simulink library "csc_tdl_thruster_dynamics_collection_lib"  (R2014b)
settings: Solver=ode45  StartTime=0.0  StopTime=10.0  RelTol=1e-3
libraries: csu_tdl_thruster_dynamics_lander_lib x26
settings Model: Creator=escrane  LastModifiedBy=mstewart

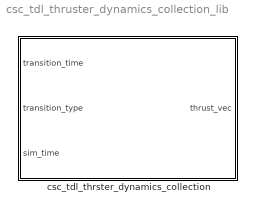
== system csc_tdl_thruster_dynamics_collection_lib ==
  csc_tdl_thrster_dynamics_collection : Subsystem
      mask Display: color('blue');text(0.05, 0.02, 'MoonEx', 'HorizontalAlignment', 'Left', 'VerticalAlignment', 'Bottom');color('red');text(0.95, 0.02, 'Autogenerated', 'HorizontalAlignment', 'Right', 'VerticalAlignment', 'Bottom');

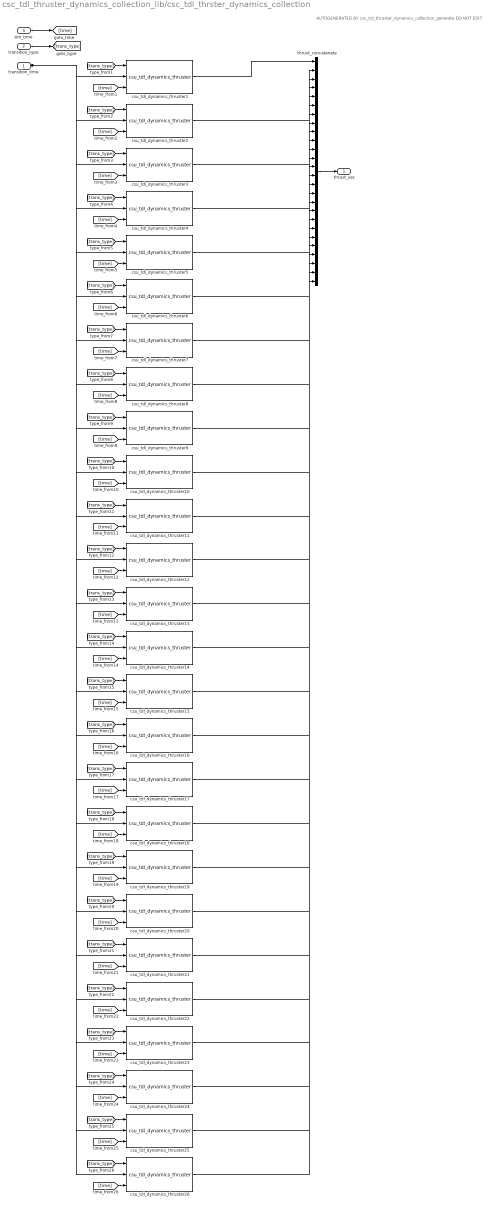
== system csc_tdl_thruster_dynamics_collection_lib/csc_tdl_thrster_dynamics_collection ==
  note: AUTOGENERATED BY csc_tdl_thruster_dynamics_collection_generate
      | DO NOT EDIT
  transition_time : Inport
  transition_type : Inport  Port=2
  sim_time : Inport  Port=3
  csu_tdl_dynamics_thruster1 : csu_tdl_thruster_dynamics_lander_lib/csu_tdl_dynamics_thruster  thruster_idx=1  num_thrusters=26  time_since_rise_lookup=tdl_thruster1_rising_lookup_time  thrust_rising_output_lookup=tdl_thruster1_rising_lookup_thrust  time_since_fall_lookup=tdl_thruster1_falling_lookup_time  thrust_falling_output_lookup=tdl_thruster1_falling_lookup_thrust  thrust_noise_mean=tdl_thruster1_thrust_noise_mean  thrust_noise_std=tdl_thruster1_thrust_noise_std  thrust_noise_seed=tdl_thruster1_thrust_noise_seed  thrust_noise_on=tdl_thruster1_thrust_noise_enable
  csu_tdl_dynamics_thruster10 : csu_tdl_thruster_dynamics_lander_lib/csu_tdl_dynamics_thruster  thruster_idx=10  num_thrusters=26  time_since_rise_lookup=tdl_thruster10_rising_lookup_time  thrust_rising_output_lookup=tdl_thruster10_rising_lookup_thrust  time_since_fall_lookup=tdl_thruster10_falling_lookup_time  thrust_falling_output_lookup=tdl_thruster10_falling_lookup_thrust  thrust_noise_mean=tdl_thruster10_thrust_noise_mean  thrust_noise_std=tdl_thruster10_thrust_noise_std  thrust_noise_seed=tdl_thruster10_thrust_noise_seed  thrust_noise_on=tdl_thruster10_thrust_noise_enable
  csu_tdl_dynamics_thruster11 : csu_tdl_thruster_dynamics_lander_lib/csu_tdl_dynamics_thruster  thruster_idx=11  num_thrusters=26  time_since_rise_lookup=tdl_thruster11_rising_lookup_time  thrust_rising_output_lookup=tdl_thruster11_rising_lookup_thrust  time_since_fall_lookup=tdl_thruster11_falling_lookup_time  thrust_falling_output_lookup=tdl_thruster11_falling_lookup_thrust  thrust_noise_mean=tdl_thruster11_thrust_noise_mean  thrust_noise_std=tdl_thruster11_thrust_noise_std  thrust_noise_seed=tdl_thruster11_thrust_noise_seed  thrust_noise_on=tdl_thruster11_thrust_noise_enable
  csu_tdl_dynamics_thruster12 : csu_tdl_thruster_dynamics_lander_lib/csu_tdl_dynamics_thruster  thruster_idx=12  num_thrusters=26  time_since_rise_lookup=tdl_thruster12_rising_lookup_time  thrust_rising_output_lookup=tdl_thruster12_rising_lookup_thrust  time_since_fall_lookup=tdl_thruster12_falling_lookup_time  thrust_falling_output_lookup=tdl_thruster12_falling_lookup_thrust  thrust_noise_mean=tdl_thruster12_thrust_noise_mean  thrust_noise_std=tdl_thruster12_thrust_noise_std  thrust_noise_seed=tdl_thruster12_thrust_noise_seed  thrust_noise_on=tdl_thruster12_thrust_noise_enable
  csu_tdl_dynamics_thruster13 : csu_tdl_thruster_dynamics_lander_lib/csu_tdl_dynamics_thruster  thruster_idx=13  num_thrusters=26  time_since_rise_lookup=tdl_thruster13_rising_lookup_time  thrust_rising_output_lookup=tdl_thruster13_rising_lookup_thrust  time_since_fall_lookup=tdl_thruster13_falling_lookup_time  thrust_falling_output_lookup=tdl_thruster13_falling_lookup_thrust  thrust_noise_mean=tdl_thruster13_thrust_noise_mean  thrust_noise_std=tdl_thruster13_thrust_noise_std  thrust_noise_seed=tdl_thruster13_thrust_noise_seed  thrust_noise_on=tdl_thruster13_thrust_noise_enable
  csu_tdl_dynamics_thruster14 : csu_tdl_thruster_dynamics_lander_lib/csu_tdl_dynamics_thruster  thruster_idx=14  num_thrusters=26  time_since_rise_lookup=tdl_thruster14_rising_lookup_time  thrust_rising_output_lookup=tdl_thruster14_rising_lookup_thrust  time_since_fall_lookup=tdl_thruster14_falling_lookup_time  thrust_falling_output_lookup=tdl_thruster14_falling_lookup_thrust  thrust_noise_mean=tdl_thruster14_thrust_noise_mean  thrust_noise_std=tdl_thruster14_thrust_noise_std  thrust_noise_seed=tdl_thruster14_thrust_noise_seed  thrust_noise_on=tdl_thruster14_thrust_noise_enable
  csu_tdl_dynamics_thruster15 : csu_tdl_thruster_dynamics_lander_lib/csu_tdl_dynamics_thruster  thruster_idx=15  num_thrusters=26  time_since_rise_lookup=tdl_thruster15_rising_lookup_time  thrust_rising_output_lookup=tdl_thruster15_rising_lookup_thrust  time_since_fall_lookup=tdl_thruster15_falling_lookup_time  thrust_falling_output_lookup=tdl_thruster15_falling_lookup_thrust  thrust_noise_mean=tdl_thruster15_thrust_noise_mean  thrust_noise_std=tdl_thruster15_thrust_noise_std  thrust_noise_seed=tdl_thruster15_thrust_noise_seed  thrust_noise_on=tdl_thruster15_thrust_noise_enable
  csu_tdl_dynamics_thruster16 : csu_tdl_thruster_dynamics_lander_lib/csu_tdl_dynamics_thruster  thruster_idx=16  num_thrusters=26  time_since_rise_lookup=tdl_thruster16_rising_lookup_time  thrust_rising_output_lookup=tdl_thruster16_rising_lookup_thrust  time_since_fall_lookup=tdl_thruster16_falling_lookup_time  thrust_falling_output_lookup=tdl_thruster16_falling_lookup_thrust  thrust_noise_mean=tdl_thruster16_thrust_noise_mean  thrust_noise_std=tdl_thruster16_thrust_noise_std  thrust_noise_seed=tdl_thruster16_thrust_noise_seed  thrust_noise_on=tdl_thruster16_thrust_noise_enable
  csu_tdl_dynamics_thruster17 : csu_tdl_thruster_dynamics_lander_lib/csu_tdl_dynamics_thruster  thruster_idx=17  num_thrusters=26  time_since_rise_lookup=tdl_thruster17_rising_lookup_time  thrust_rising_output_lookup=tdl_thruster17_rising_lookup_thrust  time_since_fall_lookup=tdl_thruster17_falling_lookup_time  thrust_falling_output_lookup=tdl_thruster17_falling_lookup_thrust  thrust_noise_mean=tdl_thruster17_thrust_noise_mean  thrust_noise_std=tdl_thruster17_thrust_noise_std  thrust_noise_seed=tdl_thruster17_thrust_noise_seed  thrust_noise_on=tdl_thruster17_thrust_noise_enable
  csu_tdl_dynamics_thruster18 : csu_tdl_thruster_dynamics_lander_lib/csu_tdl_dynamics_thruster  thruster_idx=18  num_thrusters=26  time_since_rise_lookup=tdl_thruster18_rising_lookup_time  thrust_rising_output_lookup=tdl_thruster18_rising_lookup_thrust  time_since_fall_lookup=tdl_thruster18_falling_lookup_time  thrust_falling_output_lookup=tdl_thruster18_falling_lookup_thrust  thrust_noise_mean=tdl_thruster18_thrust_noise_mean  thrust_noise_std=tdl_thruster18_thrust_noise_std  thrust_noise_seed=tdl_thruster18_thrust_noise_seed  thrust_noise_on=tdl_thruster18_thrust_noise_enable
  csu_tdl_dynamics_thruster19 : csu_tdl_thruster_dynamics_lander_lib/csu_tdl_dynamics_thruster  thruster_idx=19  num_thrusters=26  time_since_rise_lookup=tdl_thruster19_rising_lookup_time  thrust_rising_output_lookup=tdl_thruster19_rising_lookup_thrust  time_since_fall_lookup=tdl_thruster19_falling_lookup_time  thrust_falling_output_lookup=tdl_thruster19_falling_lookup_thrust  thrust_noise_mean=tdl_thruster19_thrust_noise_mean  thrust_noise_std=tdl_thruster19_thrust_noise_std  thrust_noise_seed=tdl_thruster19_thrust_noise_seed  thrust_noise_on=tdl_thruster19_thrust_noise_enable
  csu_tdl_dynamics_thruster2 : csu_tdl_thruster_dynamics_lander_lib/csu_tdl_dynamics_thruster  thruster_idx=2  num_thrusters=26  time_since_rise_lookup=tdl_thruster2_rising_lookup_time  thrust_rising_output_lookup=tdl_thruster2_rising_lookup_thrust  time_since_fall_lookup=tdl_thruster2_falling_lookup_time  thrust_falling_output_lookup=tdl_thruster2_falling_lookup_thrust  thrust_noise_mean=tdl_thruster2_thrust_noise_mean  thrust_noise_std=tdl_thruster2_thrust_noise_std  thrust_noise_seed=tdl_thruster2_thrust_noise_seed  thrust_noise_on=tdl_thruster2_thrust_noise_enable
  csu_tdl_dynamics_thruster20 : csu_tdl_thruster_dynamics_lander_lib/csu_tdl_dynamics_thruster  thruster_idx=20  num_thrusters=26  time_since_rise_lookup=tdl_thruster20_rising_lookup_time  thrust_rising_output_lookup=tdl_thruster20_rising_lookup_thrust  time_since_fall_lookup=tdl_thruster20_falling_lookup_time  thrust_falling_output_lookup=tdl_thruster20_falling_lookup_thrust  thrust_noise_mean=tdl_thruster20_thrust_noise_mean  thrust_noise_std=tdl_thruster20_thrust_noise_std  thrust_noise_seed=tdl_thruster20_thrust_noise_seed  thrust_noise_on=tdl_thruster20_thrust_noise_enable
  csu_tdl_dynamics_thruster21 : csu_tdl_thruster_dynamics_lander_lib/csu_tdl_dynamics_thruster  thruster_idx=21  num_thrusters=26  time_since_rise_lookup=tdl_thruster21_rising_lookup_time  thrust_rising_output_lookup=tdl_thruster21_rising_lookup_thrust  time_since_fall_lookup=tdl_thruster21_falling_lookup_time  thrust_falling_output_lookup=tdl_thruster21_falling_lookup_thrust  thrust_noise_mean=tdl_thruster21_thrust_noise_mean  thrust_noise_std=tdl_thruster21_thrust_noise_std  thrust_noise_seed=tdl_thruster21_thrust_noise_seed  thrust_noise_on=tdl_thruster21_thrust_noise_enable
  csu_tdl_dynamics_thruster22 : csu_tdl_thruster_dynamics_lander_lib/csu_tdl_dynamics_thruster  thruster_idx=22  num_thrusters=26  time_since_rise_lookup=tdl_thruster22_rising_lookup_time  thrust_rising_output_lookup=tdl_thruster22_rising_lookup_thrust  time_since_fall_lookup=tdl_thruster22_falling_lookup_time  thrust_falling_output_lookup=tdl_thruster22_falling_lookup_thrust  thrust_noise_mean=tdl_thruster22_thrust_noise_mean  thrust_noise_std=tdl_thruster22_thrust_noise_std  thrust_noise_seed=tdl_thruster22_thrust_noise_seed  thrust_noise_on=tdl_thruster22_thrust_noise_enable
  csu_tdl_dynamics_thruster23 : csu_tdl_thruster_dynamics_lander_lib/csu_tdl_dynamics_thruster  thruster_idx=23  num_thrusters=26  time_since_rise_lookup=tdl_thruster23_rising_lookup_time  thrust_rising_output_lookup=tdl_thruster23_rising_lookup_thrust  time_since_fall_lookup=tdl_thruster23_falling_lookup_time  thrust_falling_output_lookup=tdl_thruster23_falling_lookup_thrust  thrust_noise_mean=tdl_thruster23_thrust_noise_mean  thrust_noise_std=tdl_thruster23_thrust_noise_std  thrust_noise_seed=tdl_thruster23_thrust_noise_seed  thrust_noise_on=tdl_thruster23_thrust_noise_enable
  csu_tdl_dynamics_thruster24 : csu_tdl_thruster_dynamics_lander_lib/csu_tdl_dynamics_thruster  thruster_idx=24  num_thrusters=26  time_since_rise_lookup=tdl_thruster24_rising_lookup_time  thrust_rising_output_lookup=tdl_thruster24_rising_lookup_thrust  time_since_fall_lookup=tdl_thruster24_falling_lookup_time  thrust_falling_output_lookup=tdl_thruster24_falling_lookup_thrust  thrust_noise_mean=tdl_thruster24_thrust_noise_mean  thrust_noise_std=tdl_thruster24_thrust_noise_std  thrust_noise_seed=tdl_thruster24_thrust_noise_seed  thrust_noise_on=tdl_thruster24_thrust_noise_enable
  csu_tdl_dynamics_thruster25 : csu_tdl_thruster_dynamics_lander_lib/csu_tdl_dynamics_thruster  thruster_idx=25  num_thrusters=26  time_since_rise_lookup=tdl_thruster25_rising_lookup_time  thrust_rising_output_lookup=tdl_thruster25_rising_lookup_thrust  time_since_fall_lookup=tdl_thruster25_falling_lookup_time  thrust_falling_output_lookup=tdl_thruster25_falling_lookup_thrust  thrust_noise_mean=tdl_thruster25_thrust_noise_mean  thrust_noise_std=tdl_thruster25_thrust_noise_std  thrust_noise_seed=tdl_thruster25_thrust_noise_seed  thrust_noise_on=tdl_thruster25_thrust_noise_enable
  csu_tdl_dynamics_thruster26 : csu_tdl_thruster_dynamics_lander_lib/csu_tdl_dynamics_thruster  thruster_idx=26  num_thrusters=26  time_since_rise_lookup=tdl_thruster26_rising_lookup_time  thrust_rising_output_lookup=tdl_thruster26_rising_lookup_thrust  time_since_fall_lookup=tdl_thruster26_falling_lookup_time  thrust_falling_output_lookup=tdl_thruster26_falling_lookup_thrust  thrust_noise_mean=tdl_thruster26_thrust_noise_mean  thrust_noise_std=tdl_thruster26_thrust_noise_std  thrust_noise_seed=tdl_thruster26_thrust_noise_seed  thrust_noise_on=tdl_thruster26_thrust_noise_enable
  csu_tdl_dynamics_thruster3 : csu_tdl_thruster_dynamics_lander_lib/csu_tdl_dynamics_thruster  thruster_idx=3  num_thrusters=26  time_since_rise_lookup=tdl_thruster3_rising_lookup_time  thrust_rising_output_lookup=tdl_thruster3_rising_lookup_thrust  time_since_fall_lookup=tdl_thruster3_falling_lookup_time  thrust_falling_output_lookup=tdl_thruster3_falling_lookup_thrust  thrust_noise_mean=tdl_thruster3_thrust_noise_mean  thrust_noise_std=tdl_thruster3_thrust_noise_std  thrust_noise_seed=tdl_thruster3_thrust_noise_seed  thrust_noise_on=tdl_thruster3_thrust_noise_enable
  csu_tdl_dynamics_thruster4 : csu_tdl_thruster_dynamics_lander_lib/csu_tdl_dynamics_thruster  thruster_idx=4  num_thrusters=26  time_since_rise_lookup=tdl_thruster4_rising_lookup_time  thrust_rising_output_lookup=tdl_thruster4_rising_lookup_thrust  time_since_fall_lookup=tdl_thruster4_falling_lookup_time  thrust_falling_output_lookup=tdl_thruster4_falling_lookup_thrust  thrust_noise_mean=tdl_thruster4_thrust_noise_mean  thrust_noise_std=tdl_thruster4_thrust_noise_std  thrust_noise_seed=tdl_thruster4_thrust_noise_seed  thrust_noise_on=tdl_thruster4_thrust_noise_enable
  csu_tdl_dynamics_thruster5 : csu_tdl_thruster_dynamics_lander_lib/csu_tdl_dynamics_thruster  thruster_idx=5  num_thrusters=26  time_since_rise_lookup=tdl_thruster5_rising_lookup_time  thrust_rising_output_lookup=tdl_thruster5_rising_lookup_thrust  time_since_fall_lookup=tdl_thruster5_falling_lookup_time  thrust_falling_output_lookup=tdl_thruster5_falling_lookup_thrust  thrust_noise_mean=tdl_thruster5_thrust_noise_mean  thrust_noise_std=tdl_thruster5_thrust_noise_std  thrust_noise_seed=tdl_thruster5_thrust_noise_seed  thrust_noise_on=tdl_thruster5_thrust_noise_enable
  csu_tdl_dynamics_thruster6 : csu_tdl_thruster_dynamics_lander_lib/csu_tdl_dynamics_thruster  thruster_idx=6  num_thrusters=26  time_since_rise_lookup=tdl_thruster6_rising_lookup_time  thrust_rising_output_lookup=tdl_thruster6_rising_lookup_thrust  time_since_fall_lookup=tdl_thruster6_falling_lookup_time  thrust_falling_output_lookup=tdl_thruster6_falling_lookup_thrust  thrust_noise_mean=tdl_thruster6_thrust_noise_mean  thrust_noise_std=tdl_thruster6_thrust_noise_std  thrust_noise_seed=tdl_thruster6_thrust_noise_seed  thrust_noise_on=tdl_thruster6_thrust_noise_enable
  csu_tdl_dynamics_thruster7 : csu_tdl_thruster_dynamics_lander_lib/csu_tdl_dynamics_thruster  thruster_idx=7  num_thrusters=26  time_since_rise_lookup=tdl_thruster7_rising_lookup_time  thrust_rising_output_lookup=tdl_thruster7_rising_lookup_thrust  time_since_fall_lookup=tdl_thruster7_falling_lookup_time  thrust_falling_output_lookup=tdl_thruster7_falling_lookup_thrust  thrust_noise_mean=tdl_thruster7_thrust_noise_mean  thrust_noise_std=tdl_thruster7_thrust_noise_std  thrust_noise_seed=tdl_thruster7_thrust_noise_seed  thrust_noise_on=tdl_thruster7_thrust_noise_enable
  csu_tdl_dynamics_thruster8 : csu_tdl_thruster_dynamics_lander_lib/csu_tdl_dynamics_thruster  thruster_idx=8  num_thrusters=26  time_since_rise_lookup=tdl_thruster8_rising_lookup_time  thrust_rising_output_lookup=tdl_thruster8_rising_lookup_thrust  time_since_fall_lookup=tdl_thruster8_falling_lookup_time  thrust_falling_output_lookup=tdl_thruster8_falling_lookup_thrust  thrust_noise_mean=tdl_thruster8_thrust_noise_mean  thrust_noise_std=tdl_thruster8_thrust_noise_std  thrust_noise_seed=tdl_thruster8_thrust_noise_seed  thrust_noise_on=tdl_thruster8_thrust_noise_enable
  csu_tdl_dynamics_thruster9 : csu_tdl_thruster_dynamics_lander_lib/csu_tdl_dynamics_thruster  thruster_idx=9  num_thrusters=26  time_since_rise_lookup=tdl_thruster9_rising_lookup_time  thrust_rising_output_lookup=tdl_thruster9_rising_lookup_thrust  time_since_fall_lookup=tdl_thruster9_falling_lookup_time  thrust_falling_output_lookup=tdl_thruster9_falling_lookup_thrust  thrust_noise_mean=tdl_thruster9_thrust_noise_mean  thrust_noise_std=tdl_thruster9_thrust_noise_std  thrust_noise_seed=tdl_thruster9_thrust_noise_seed  thrust_noise_on=tdl_thruster9_thrust_noise_enable
  thrust_concatenate : Concatenate  NumInputs=26
  thrust_vec : Outport
  wires:
  sim_time/1 -> [time]
  transition_type/1 -> [trans_type]
  thrust_concatenate/1 -> thrust_vec/1
  [time] -> csu_tdl_dynamics_thruster1/3
  [trans_type] -> csu_tdl_dynamics_thruster1/1
  csu_tdl_dynamics_thruster1/1 -> thrust_concatenate/1
  [time] -> csu_tdl_dynamics_thruster2/3
  [trans_type] -> csu_tdl_dynamics_thruster2/1
  csu_tdl_dynamics_thruster2/1 -> thrust_concatenate/2
  [time] -> csu_tdl_dynamics_thruster3/3
  [trans_type] -> csu_tdl_dynamics_thruster3/1
  csu_tdl_dynamics_thruster3/1 -> thrust_concatenate/3
  [time] -> csu_tdl_dynamics_thruster4/3
  [trans_type] -> csu_tdl_dynamics_thruster4/1
  csu_tdl_dynamics_thruster4/1 -> thrust_concatenate/4
  [time] -> csu_tdl_dynamics_thruster5/3
  [trans_type] -> csu_tdl_dynamics_thruster5/1
  csu_tdl_dynamics_thruster5/1 -> thrust_concatenate/5
  [time] -> csu_tdl_dynamics_thruster6/3
  [trans_type] -> csu_tdl_dynamics_thruster6/1
  csu_tdl_dynamics_thruster6/1 -> thrust_concatenate/6
  [time] -> csu_tdl_dynamics_thruster7/3
  [trans_type] -> csu_tdl_dynamics_thruster7/1
  csu_tdl_dynamics_thruster7/1 -> thrust_concatenate/7
  [time] -> csu_tdl_dynamics_thruster8/3
  [trans_type] -> csu_tdl_dynamics_thruster8/1
  csu_tdl_dynamics_thruster8/1 -> thrust_concatenate/8
  [time] -> csu_tdl_dynamics_thruster9/3
  [trans_type] -> csu_tdl_dynamics_thruster9/1
  csu_tdl_dynamics_thruster9/1 -> thrust_concatenate/9
  [time] -> csu_tdl_dynamics_thruster10/3
  [trans_type] -> csu_tdl_dynamics_thruster10/1
  csu_tdl_dynamics_thruster10/1 -> thrust_concatenate/10
  [time] -> csu_tdl_dynamics_thruster11/3
  [trans_type] -> csu_tdl_dynamics_thruster11/1
  csu_tdl_dynamics_thruster11/1 -> thrust_concatenate/11
  [time] -> csu_tdl_dynamics_thruster12/3
  [trans_type] -> csu_tdl_dynamics_thruster12/1
  csu_tdl_dynamics_thruster12/1 -> thrust_concatenate/12
  [time] -> csu_tdl_dynamics_thruster13/3
  [trans_type] -> csu_tdl_dynamics_thruster13/1
  csu_tdl_dynamics_thruster13/1 -> thrust_concatenate/13
  [time] -> csu_tdl_dynamics_thruster14/3
  [trans_type] -> csu_tdl_dynamics_thruster14/1
  csu_tdl_dynamics_thruster14/1 -> thrust_concatenate/14
  [time] -> csu_tdl_dynamics_thruster15/3
  [trans_type] -> csu_tdl_dynamics_thruster15/1
  csu_tdl_dynamics_thruster15/1 -> thrust_concatenate/15
  [time] -> csu_tdl_dynamics_thruster16/3
  [trans_type] -> csu_tdl_dynamics_thruster16/1
  csu_tdl_dynamics_thruster16/1 -> thrust_concatenate/16
  [time] -> csu_tdl_dynamics_thruster17/3
  [trans_type] -> csu_tdl_dynamics_thruster17/1
  csu_tdl_dynamics_thruster17/1 -> thrust_concatenate/17
  [time] -> csu_tdl_dynamics_thruster18/3
  [trans_type] -> csu_tdl_dynamics_thruster18/1
  csu_tdl_dynamics_thruster18/1 -> thrust_concatenate/18
  [time] -> csu_tdl_dynamics_thruster19/3
  [trans_type] -> csu_tdl_dynamics_thruster19/1
  csu_tdl_dynamics_thruster19/1 -> thrust_concatenate/19
  [time] -> csu_tdl_dynamics_thruster20/3
  [trans_type] -> csu_tdl_dynamics_thruster20/1
  csu_tdl_dynamics_thruster20/1 -> thrust_concatenate/20
  [time] -> csu_tdl_dynamics_thruster21/3
  [trans_type] -> csu_tdl_dynamics_thruster21/1
  csu_tdl_dynamics_thruster21/1 -> thrust_concatenate/21
  [time] -> csu_tdl_dynamics_thruster22/3
  [trans_type] -> csu_tdl_dynamics_thruster22/1
  csu_tdl_dynamics_thruster22/1 -> thrust_concatenate/22
  [time] -> csu_tdl_dynamics_thruster23/3
  [trans_type] -> csu_tdl_dynamics_thruster23/1
  csu_tdl_dynamics_thruster23/1 -> thrust_concatenate/23
  [time] -> csu_tdl_dynamics_thruster24/3
  [trans_type] -> csu_tdl_dynamics_thruster24/1
  csu_tdl_dynamics_thruster24/1 -> thrust_concatenate/24
  [time] -> csu_tdl_dynamics_thruster25/3
  [trans_type] -> csu_tdl_dynamics_thruster25/1
  csu_tdl_dynamics_thruster25/1 -> thrust_concatenate/25
  [time] -> csu_tdl_dynamics_thruster26/3
  [trans_type] -> csu_tdl_dynamics_thruster26/1
  csu_tdl_dynamics_thruster26/1 -> thrust_concatenate/26
  transition_time/1 -> csu_tdl_dynamics_thruster26/2, csu_tdl_dynamics_thruster25/2, csu_tdl_dynamics_thruster24/2, csu_tdl_dynamics_thruster23/2, csu_tdl_dynamics_thruster22/2, csu_tdl_dynamics_thruster21/2, csu_tdl_dynamics_thruster20/2, csu_tdl_dynamics_thruster19/2, csu_tdl_dynamics_thruster18/2, csu_tdl_dynamics_thruster17/2, csu_tdl_dynamics_thruster16/2, csu_tdl_dynamics_thruster15/2, csu_tdl_dynamics_thruster14/2, csu_tdl_dynamics_thruster13/2, csu_tdl_dynamics_thruster12/2, csu_tdl_dynamics_thruster11/2, csu_tdl_dynamics_thruster10/2, csu_tdl_dynamics_thruster9/2, csu_tdl_dynamics_thruster8/2, csu_tdl_dynamics_thruster7/2, csu_tdl_dynamics_thruster6/2, csu_tdl_dynamics_thruster5/2, csu_tdl_dynamics_thruster4/2, csu_tdl_dynamics_thruster3/2, csu_tdl_dynamics_thruster2/2, csu_tdl_dynamics_thruster1/2
